simulink library "tos_lib"  (Simulink 7.4)
settings: Solver=ode45  SolverMode=SingleTasking  StartTime=0.0  StopTime=10.0  RelTol=1e-3
values from neighbouring files (symbols this model uses):
  baud = 115200    [test.m]
  com = '/dev/ttyACM0,output2.txt'    [test.m]
  fTf = 0.5    [test.m]
  fTl = 0.5    [test.m]
  fTt = 0.5    [test.m]
  Ts = 0.02    [test.m]
settings Model: Creator=gvallabh  LastModifiedBy=tom

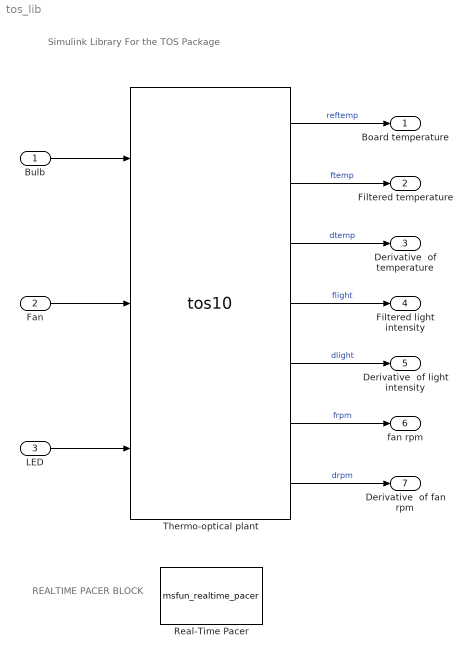
== system tos_lib ==
  note: Simulink Library For the TOS Package
  note: REALTIME
      | PACER
      | BLOCK
  Bulb : Inport  OutDataType=fixdt(1, 16)  OutScaling=2^0
  Fan : Inport  Port=2  OutDataType=fixdt(1, 16)  OutScaling=2^0
  LED : Inport  Port=3  OutDataType=fixdt(1, 16)  OutScaling=2^0
  Real-Time Pacer : M-S-Function  FunctionName=msfun_realtime_pacer  Parameters=simTimePerRealTime  mask(RealTime_Pacer){simTimePerRealTime=1}
      mask prompts: simTimePerRealTime "Speedup (Simulation Time / Real Time):"
      mask help:
      | Slow down a simulation to track real (i.e., wall clock) elapsed time.
      |
      | "Speedup" specifies the ratio between simulation time and real time
      |  Speedup = N => N sec. of simulation time per sec. of real time
      |  Speedup can be fractional (e.g., 0.5, 1.3).
      |  Speedup = inf => allow simulation to run at full speed
      |
      | Click on the Help button for details.
      mask Help: web('realtime_pacer_help.html', '-helpbrowser')
      mask Display: fprintf('Real-Time Pacer\nSpeedup = %g', simTimePerRealTime)
  Thermo-optical plant : M-S-Function  FunctionName=tos10  Parameters=Ts,com,baud,fTt,fTl,fTf
  Board temperature : Outport  OutDataType=fixdt(1, 16)  OutScaling=2^0
  Filtered temperature : Outport  Port=2  OutDataType=fixdt(1, 16)  OutScaling=2^0
  Derivative  of temperature : Outport  Port=3  OutDataType=fixdt(1, 16)  OutScaling=2^0
  Filtered light intensity : Outport  Port=4  OutDataType=fixdt(1, 16)  OutScaling=2^0
  Derivative  of light intensity : Outport  Port=5  OutDataType=fixdt(1, 16)  OutScaling=2^0
  fan rpm : Outport  Port=6  OutDataType=fixdt(1, 16)  OutScaling=2^0
  Derivative  of fan rpm : Outport  Port=7  OutDataType=fixdt(1, 16)  OutScaling=2^0
  wires:
  Thermo-optical plant/1 -> Board temperature/1  "reftemp"
  Thermo-optical plant/2 -> Filtered temperature/1  "ftemp"
  Thermo-optical plant/3 -> Derivative  of temperature/1  "dtemp"
  Thermo-optical plant/4 -> Filtered light intensity/1  "flight"
  Thermo-optical plant/5 -> Derivative  of light intensity/1  "dlight"
  Thermo-optical plant/6 -> fan rpm/1  "frpm"
  Thermo-optical plant/7 -> Derivative  of fan rpm/1  "drpm"
  Bulb/1 -> Thermo-optical plant/1
  Fan/1 -> Thermo-optical plant/2
  LED/1 -> Thermo-optical plant/3
